simulink model "MBD_Sources_Signal_Bulider_Block"  (R2021b)
settings: Solver=FixedStepDiscrete  StartTime=0.0  StopTime=10.0  FixedStep=0.01  RelTol=1e-3
undefined symbols (not defined in the file or in its folder): sigbuilder_block
settings Model: Creator=waleed.elshemy  LastModifiedBy=ADMIN

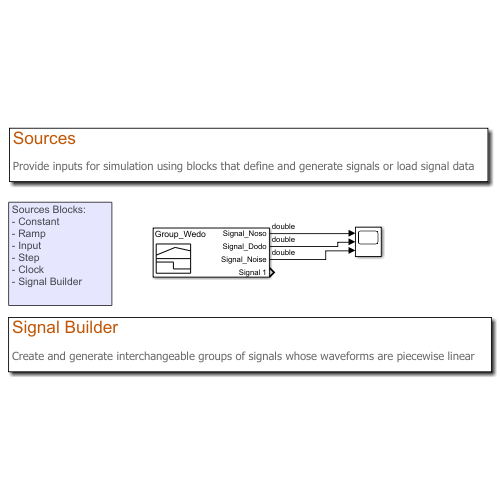
[thumbnail: Simulink's stored preview of the top-level diagram]
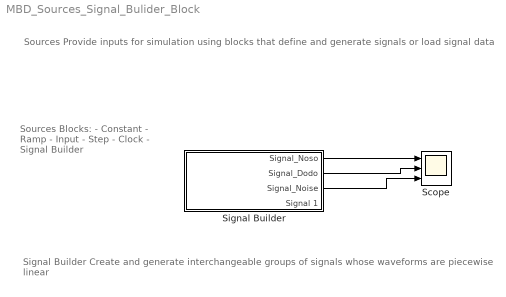
== system MBD_Sources_Signal_Bulider_Block ==
  note: Signal Builder
      | Create and generate interchangeable groups of signals whose waveforms are piecewise linear
  note: Sources
      | Provide inputs for simulation using blocks that define and generate signals or load signal data
  note: Sources Blocks:
      | - Constant
      | - Ramp
      | - Input
      | - Step
      | - Clock
      | - Signal Builder
  Scope : Scope  NumInputPorts=3
  Signal Builder : Subsystem  Tag=STV Subsys  LoadFcn=sigbuilder_block('load');  StartFcn=sigbuilder_block('start');  StopFcn=sigbuilder_block('stop');  ClipboardFcn=sigbuilder_block('clipboard');  mask(Sigbuilder block){tuvar=[0:10]}
      mask help: Simulink:masks:SigbuilderBlock_MD
      mask init:
      | if ~strcmp(get_param(bdroot(gcbh),'SimulationStatus'),'stopped') tuvar = sigbuilder_block('maskInit'); end
      settings: CopyFcn=sigbuilder_block('copy');  DeleteFcn=sigbuilder_block('delete');  ModelCloseFcn=sigbuilder_block('modelClose');  PreSaveFcn=sigbuilder_block('preSave');  PauseFcn=sigbuilder_block('pause');  ContinueFcn=sigbuilder_block('continue');  NameChangeFcn=sigbuilder_block('namechange');  OpenFcn=sigbuilder_block('open',[7 94.5 522.5 360.5 ]);  CloseFcn=sigbuilder_block('close');
      mask Display: plot(0, 0, 100, 100,[2, 2, 32, 32, 2], [68, 8, 8, 68, 68],[32, 2], [38, 38], [32, 19, 2],[53, 60, 44], [32, 17, 17, 2],[16, 16, 31, 31]);txt = getActiveGroup(gcbh);text(2, 100, txt,'verticalAlignment', 'top');
  wires:
  Signal Builder/1(Signal_Noso) -> Scope/1
  Signal Builder/2(Signal_Dodo) -> Scope/2
  Signal Builder/3(Signal_Noise) -> Scope/3

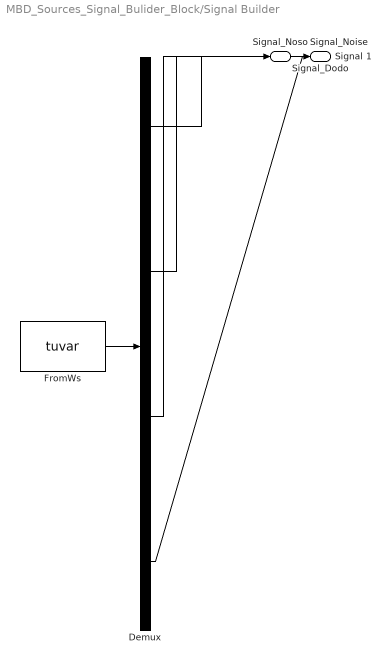
== system MBD_Sources_Signal_Bulider_Block/Signal Builder ==
  Demux : Demux  Tag=STV Demux
      settings: DisplayOption=none
  FromWs : FromWorkspace  Tag=STV FromWs  VariableName=tuvar
      SigBuilderData=|
      | common.afterFinalStr = 'Extrapolate'
      | common.sampleTime = 0
      | dataSet.timeRange = [0 10]
      | dataSet.name = 'Group_Wedo'
      | sbobj.Groups.Name = 'Group_Wedo'
      | sbobj.Groups.Signals(1).Name = 'Signal_Noso'
      | sbobj.Groups.Signals(1).XData = [0 2 3.96 6 6 10]
      | sbobj.Groups.Signals(1).YData = [0 0.3 1 1 0 0]
      | sbobj.Groups.Signals(2).Name = 'Signal_Dodo'
      | sbobj.Groups.Signals(2).XData = [0 0.1 0.2 0.3 0.4 0.5 0.6 0.7 0.8 0.9 1 1.1 1.2 1.3 1.4 1.5 1.6 1.7 1.8 1.9 2 2.1 2.2 2.3 2.4 2.5 2.6 2.7 2.8 2.9 3 3.1 3.2 3.3 3.4 3.5 3.6 3.7 3.8 3.9 4 4.1 4.2 4.3 4.4 4.5 4.6 4.7 4.8 4.9 5 5.1 5.2 5.3 5.4 5.5 5.6 5.7 5.8 5.9 6 6.1 6.2 6.3 6.4 6.5 6.6 6.7 6.8 6.9 7 7.1 7.2 7.3 7.4 7.5 7.6 7.7 7.8 7.9 10]
      | sbobj.Groups.Signals(2).YData = [0 0.0998334166468 0.198669330795 0.295520206661 0.389418342309 0.479425538604 0.564642473395 0.644217687238 0.7173560909 0.783326909627 0.841470984808 0.891207360061 0.932039085967 0.963558185417 0.985449729988 0.997494986604 0.999573603042 0.991664810452 0.973847630878 0.946300087687 0.909297426826 0.863209366649 0.80849640382 0.745705212177 0.675463180551 0.598472144104 0.515501371821 0.427379880234 0.334988150156 0.239249329214 0.14112000806 0.0415806624333 -0.0583741434276 -0.157745694143 -0.255541102027 -0.35078322769 -0.442520443295 -0.529836140908 -0.611857890943 -0.687766159184 -0.756802495308 -0.818277111064 -0.871575772414 -0.916165936749 -0.95160207389 -0.977530117665 -0.993691003633 -0.999923257564 -0.996164608836 -0.982452612624 -0.958924274663 -0.925814682328 -0.88345465572 -0.832267442224 -0.772764487556 -0.70554032557 -0.631266637872 -0.550685542598 -0.464602179414 -0.37387666483 -0.279415498199 -0.182162504272 -0.0830894028175 0.0168139004843 0.11654920485 0.215119988088 0.311541363513 0.404849920617 0.494113351139 0.578439764388 0.656986598719 0.728969040126 0.793667863849 0.850436620629 0.898708095812 0.937999976775 0.967919672031 0.988168233877 0.998543345375 0.99894134184 0.99894134184]
      | sbobj.Groups.Signals(3).Name = 'Signal_Noise'
      | sbobj.Groups.Signals(3).XData = [0 1 1 2 2 3 3 4 4 5 5 6 6 7 7 10]
      | sbobj.Groups.Signals(3).YData = [0 2 0 2 0 2 0 2 0 2 0 2 0 2 0 0]
      | sbobj.Groups.Signals(4).Name = 'Signal 1'
      | sbobj.Groups.Signals(4).XData = [0 5 5 10]
      | sbobj.Groups.Signals(4).YData = [0 0 2.5 2.5]
  Signal_Noso : Outport  Tag=STV Outport
  Signal_Dodo : Outport  Tag=STV Outport  Port=2
  Signal_Noise : Outport  Tag=STV Outport  Port=3
  Signal 1 : Outport  Tag=STV Outport  Port=4
  wires:
  Demux/1 -> Signal_Noso/1
  FromWs/1 -> Demux/1
  Demux/2 -> Signal_Dodo/1
  Demux/3 -> Signal_Noise/1
  Demux/4 -> Signal 1/1
